simulink subsystem "Piero_ModelZ"  (R2023b)
settings: Solver=VariableStepAuto  StartTime=0.0  StopTime=10.0  RelTol=1e-3
settings Model: Creator=Carlos  LastModifiedBy=Carlos

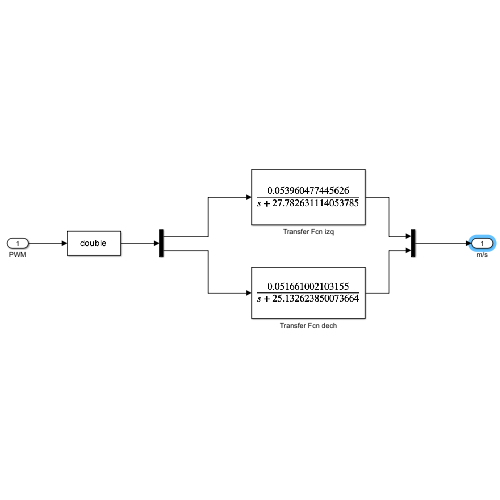
[thumbnail: Simulink's stored preview of the top-level diagram]
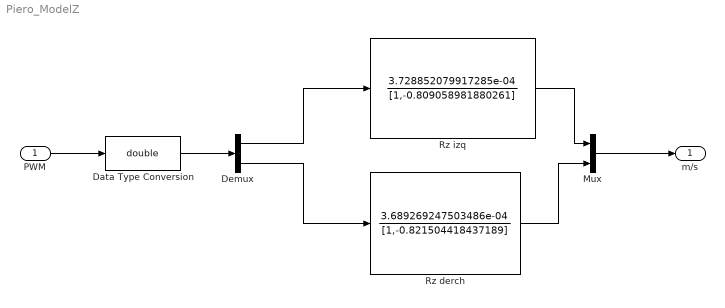
== system Piero_ModelZ ==
  PWM : Inport
  Data Type Conversion : DataTypeConversion  OutDataTypeStr=double  SaturateOnIntegerOverflow=off  RndMeth=Floor
  Demux : Demux  Outputs=2
  Mux : Mux  Inputs=2
  Rz derch : DiscreteFilter  Numerator=3.689269247503486e-04  Denominator=[1,-0.821504418437189]
  Rz izq : DiscreteFilter  Numerator=3.728852079917285e-04  Denominator=[1,-0.809058981880261]
  m/s : Outport
  wires:
  Mux/1 -> m/s/1
  Demux/1 -> Rz izq/1
  Demux/2 -> Rz derch/1
  Rz izq/1 -> Mux/1
  Rz derch/1 -> Mux/2
  Data Type Conversion/1 -> Demux/1
  PWM/1 -> Data Type Conversion/1
